simulink model "Problem5"  (R2020b)
settings: Solver=VariableStepAuto  StartTime=0.0  StopTime=100  RelTol=1e-3
model workspace (MAT data in the model file):
  C = Simulink.Parameter
  C.Value = 1e-05
  C.DataType = 'auto'
  C.Dimensions = [1 1]
  R = Simulink.Parameter
  R.Value = 10
  R.DataType = 'auto'
  R.Dimensions = [1 1]
libraries: simulink x2
settings Model: OrderedModelArguments=off  Creator=hp  LastModifiedBy=hp

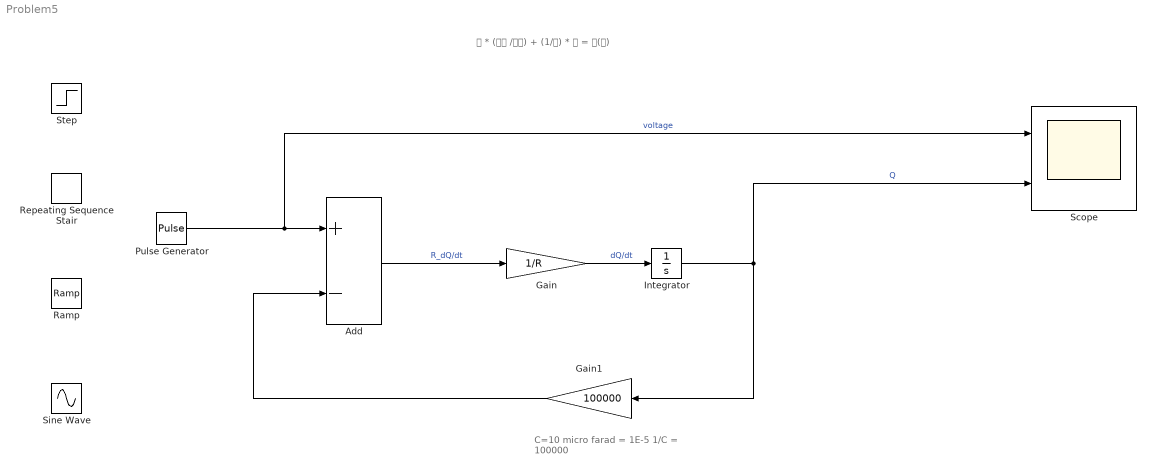
== system Problem5 ==
  note: C=10 micro farad = 1E-5
      | 1/C = 100000
  note: 𝑅 * (𝑑𝑄 /𝑑𝑡) + (1/𝐶) * 𝑄 = 𝐸(𝑡)
  Add : Sum  Inputs=+-
  Gain : Gain  Gain=1/R
  Gain1 : Gain  Gain=100000
  Integrator : Integrator  InitialCondition=4
  Pulse Generator : DiscretePulseGenerator  PulseType=Time based  Period=10  PulseWidth=5
  Ramp : simulink/Sources/Ramp  slope=1  start=0  InitialOutput=0
  Repeating Sequence Stair : simulink/Sources/Repeating Sequence Stair  OutValues=[3 1 4 2 1].'  tsamp=-1  OutMin=[]  OutMax=[]  OutDataTypeStr=double  OutputDataTypeScalingMode=double  OutDataType=fixdt(0,8)  ConRadixGroup=Best Precision: Vector-wise  OutScaling=2^-12
  Scope : Scope  NumInputPorts=2
  Sine Wave : Sin  SampleTime=0
  Step : Step  SampleTime=0
  wires:
  Pulse Generator/1 -> Scope/1, Add/1  "voltage"
  Add/1 -> Gain/1  "R_dQ/dt"
  Gain/1 -> Integrator/1  "dQ/dt"
  Integrator/1 -> Gain1/1, Scope/2  "Q"
  Gain1/1 -> Add/2
